simulink model "mpu6050 Simulink"  (R2025b)
settings: Solver=VariableStepAuto  StartTime=0.0  StopTime=10.0  RelTol=1e-3
PreLoadFcn:
  | Parameters_Flight_Firmware
undefined symbols (not defined in the file): Liftoff_threshold, threshold_sigma, Time
libraries: arduinolib x2, arduinosensorlib x1

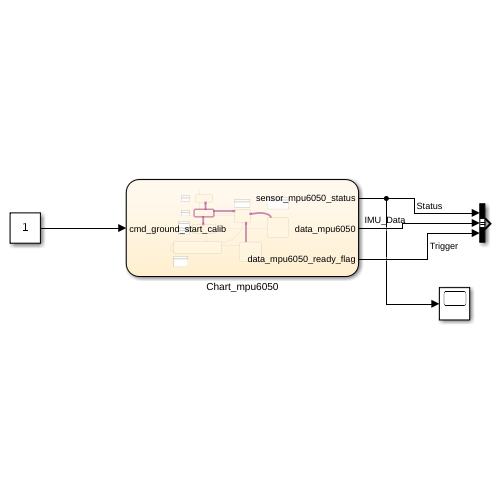
[thumbnail: Simulink's stored preview of the top-level diagram]
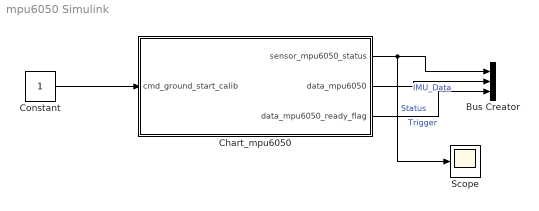
== system mpu6050 Simulink ==
  Bus Creator : BusCreator  Inputs=3
  Chart_mpu6050 : Stateflow chart  TreatAsAtomicUnit=on
  Constant : Constant
  Scope : Scope
  wires:
  Constant/1 -> Chart_mpu6050/1(cmd_ground_start_calib)
  Chart_mpu6050/1(sensor_mpu6050_status) -> Scope/1, Bus Creator/1  "Status"
  Chart_mpu6050/2(data_mpu6050) -> Bus Creator/2  "IMU_Data"
  Chart_mpu6050/3(data_mpu6050_ready_flag) -> Bus Creator/3  "Trigger"

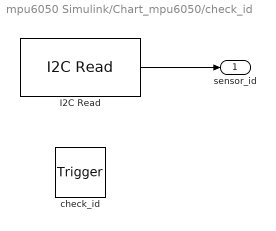
== system mpu6050 Simulink/Chart_mpu6050/check_id ==
  check_id : TriggerPort  TriggerType=function-call  VariantControl=(inherit)
      settings: CopyFcn=Stateflow.SLINSF.SimulinkMan.removeBlockPreDeleteFcn  PreDeleteFcn=Stateflow.SLINSF.SimulinkMan.unsafePredeleteFcn
  I2C Read : arduinolib/I2C Read  I2CModule=0  Mode=Master  SlaveAddress=0X68  SlaveByteOrder=BigEndian  Direction=Receiver  RegisterAddressMode=on  RegisterAddress=0X75  SlaveDataType=uint8  DataLength=1  NoAck=off  RepeatedStart=off  OutputStatus=off  blockPlatform=ARDUINO  SampleTime=-1
  sensor_id : Outport
  wires:
  I2C Read/1 -> sensor_id/1

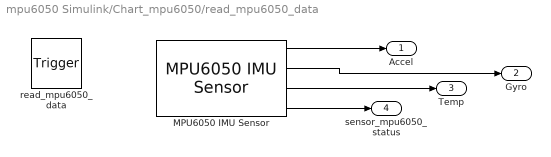
== system mpu6050 Simulink/Chart_mpu6050/read_mpu6050_data ==
  read_mpu6050_data : TriggerPort  TriggerType=function-call  VariantControl=(inherit)
      settings: CopyFcn=Stateflow.SLINSF.SimulinkMan.removeBlockPreDeleteFcn  PreDeleteFcn=Stateflow.SLINSF.SimulinkMan.unsafePredeleteFcn
  MPU6050 IMU Sensor : arduinosensorlib/MPU6050 IMU Sensor  I2CModule=0  SlaveAddress=0x68  Accel=on  AngularRate=on  Temperature=on  Status=on  Timestamp=off  EulerAngles=off  Quat=off  AccelRange=16G  GyroRange=2000 dps  DmpOdr=200 Hz  Dlpf=Accelerometer: 44Hz, Gyroscope: 42Hz  spf=1  SampleTime=-1  QueueSizeFactor=1
  Accel : Outport  OutDataTypeStr=double  PortDimensions=3
  Gyro : Outport  Port=2  OutDataTypeStr=double  PortDimensions=3
  Temp : Outport  Port=3  OutDataTypeStr=double  PortDimensions=1
  sensor_mpu6050_status : Outport  Port=4  OutDataTypeStr=uint8  PortDimensions=1
  wires:
  MPU6050 IMU Sensor/1 -> Accel/1
  MPU6050 IMU Sensor/2 -> Gyro/1
  MPU6050 IMU Sensor/3 -> Temp/1
  MPU6050 IMU Sensor/4 -> sensor_mpu6050_status/1

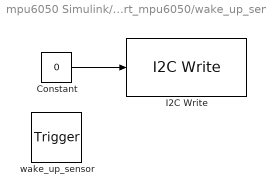
== system mpu6050 Simulink/Chart_mpu6050/wake_up_sensor ==
  wake_up_sensor : TriggerPort  TriggerType=function-call  VariantControl=(inherit)
      settings: CopyFcn=Stateflow.SLINSF.SimulinkMan.removeBlockPreDeleteFcn  PreDeleteFcn=Stateflow.SLINSF.SimulinkMan.unsafePredeleteFcn
  Constant : Constant  Value=0
  I2C Write : arduinolib/I2C Write  I2CModule=0  Mode=Master  SlaveAddress=0x68  SlaveByteOrder=BigEndian  Direction=Transmitter  RegisterAddressMode=on  RegisterAddress=0x6B  SlaveDataType=uint8  DataLength=1  NoAck=off  RepeatedStart=off  OutputStatus=off  blockPlatform=ARDUINO
  wires:
  Constant/1 -> I2C Write/1

== stateflow chart mpu6050 Simulink/Chart_mpu6050 ==
  state Power_on
    // Inizializza porte I2C
    entry: wake_up_sensor();
    delay_counter = 0;
    calib_done = false;
    during: delay_counter++;
  state wake_up_sensor [function]
  state [Accel, Gyro, Temp, sensor_mpu6050_status] = read_mpu6050_data [function]
  state Fault
    system_ready = false;
    entry: sensor_mpu6050_status = -1; // fault identity check - calibrazione fallita - Errore/Recupero
    during:
    data_mpu6050[0] = -999;
    data_mpu6050[1] = -999;
    data_mpu6050[2] = -999;
    data_mpu6050[3] = -999;
    data_mpu6050[4] = -999;
    data_mpu6050[5] = -999;
  state Sanity_Check
    entry: id_val = check_id();
    sensor_mpu6050_status = 0; // Verifica identità sensore
  state sensor_id = check_id [function]
  state Data_mpu6050_Acquisition_Raw
    entry: sensor_mpu6050_status = 3; // Sensore non calibrato - dati raw(dati grezzi)
    during: [Accel, Gyro, Temp, sensor_mpu6050_status] = read_mpu6050_data(); // Chiamata alla funzione che aggiorna le variabili locali-output per leggere i dati Raw
    // Assegnazione ai 7 slot del vettore data_mpu6050
    // Accelerazione Raw
    data_mpu6050[0] = Accel[0];
    data_mpu6050[1] = Accel[1];
    data_mpu6050[2] = Accel[2];
    // Giroscopio Raw
    data_mpu6050[3] = Gyro[0];
    data_mpu6050[4] = Gyro[1];
    data_mpu6050[5] = Gyro[2];
    // Stato Sensore mpu6050
    data_mpu6050[6] = sensor_mpu6050_status;
    data_mpu6050_ready_flag = true; // Alza il flag per il logger - via libera per la registrazione dei dati su SD
    exit: data_mpu6050_ready_flag = false; // Abbassa il flag quando esci da Data_mpu6050_Acquisition
  state Standby
    entry: system_ready = true; //Stato di attesa
    during: [Accel, Gyro, Temp, sensor_mpu6050_status] = read_mpu6050_data(); // Funzione che legge i dati grezzi dal sensore
    vibration = calc_vibration(Accel); // Calcolo la vibrazione dovuta all'accelerazione
    Az = accel_z(Accel); // Estraggo componente Z di Accel
  state Calibrating
    entry: sensor_mpu6050_status = 1; // Calibrazione del Sensore in Corso
    Reset = 1; // Al primo ingresso resettiamo la funzione Reset
    during: [Accel, Gyro, Temp, sensor_mpu6050_status] = read_mpu6050_data(); // Funzione che legge i dati grezzi dal sensore
    [mean_val, sigma, calib_done, under_threshold] = calib(Accel, Gyro, Reset, threshold_sigma)
    Reset = 0; // Dopo il primo ciclo mettiamo a 0 per continuare l'accumulo
    // Alla fine variabile calibration_done = true e mean_val == bias_val
  state Data_mpu6050_Acquisition
    entry: sensor_mpu6050_status = 2; // Stato Operativo - dati calibrati pronti per logging
    during: [Accel, Gyro, Temp, sensor_mpu6050_status] = read_mpu6050_data(); // Chiamata alla funzione che aggiorna le variabili locali-output per leggere i dati Raw
    // Assegnazione ai 7 slot del vettore data_mpu6050 sottraendo lo Zero-Bias
    // Accelerazione corretta
    data_mpu6050[0] = Accel[0] - bias_val[0];
    data_mpu6050[1] = Accel[1] - bias_val[1];
    data_mpu6050[2] = Accel[2] - bias_val[2];
    // Giroscopio corretta
    data_mpu6050[3] = Gyro[0] - bias_val[3];
    data_mpu6050[4] = Gyro[1] - bias_val[4];
    data_mpu6050[5] = Gyro[2] - bias_val[5];
    // Stato Sensore mpu6050
    data_mpu6050[6] = sensor_mpu6050_status;
    data_mpu6050_ready_flag = true; // Alza il flag per il logger - via libera per la registrazione dei dati su SD
    exit: data_mpu6050_ready_flag = false; // Abbassa il flag quando esci da Data_mpu6050_Acquisition
  (default) -> Power_on : {fail_count = 0;}
  Power_on -> Sanity_Check : [delay_counter >= 100]{fail_count = 0;}
  Sanity_Check -> Power_on [order 2] : [id_val != 104 && fail_count < 5] {fail_count = fail_count + 1;}
  Sanity_Check -> Fault [order 3] : [id_val != 104]
  Data_mpu6050_Acquisition -> Fault : [!recovery(id_val, sensor_mpu6050_status)]
  Fault -> Sanity_Check [order 1] : [fail_count < 100]{fail_count++;}
  Data_mpu6050_Acquisition_Raw -> Fault : [!recovery(id_val, sensor_mpu6050_status)]
  Fault -> Sanity_Check [order 2] : [fail_count >= 100]{fail_count = 0;}
  Sanity_Check -> Standby [order 1] : [id_val == 104]{fail_count = 0;}
  Calibrating -> Fault [order 2] : [check_id() != 104]
  Standby -> Data_mpu6050_Acquisition_Raw [order 2] : [duration(Az > Liftoff_threshold) > Time]
  Standby -> Calibrating [order 1] : [cmd_ground_start_calib == 1 && duration(vibration < Liftoff_threshold) > Time]
  Calibrating -> Calibrating [order 3] : [calib_done && !under_threshold]{Reset = 1;}
  Calibrating -> Data_mpu6050_Acquisition [order 1] : [calib_done && under_threshold]{bias_val = mean_val;}
  data: value_id function_input double; status function_input double; sanity_check function_output boolean; Accel function_output double size=3; Gyro function_output double size=3; Temp function_output double size=1; sensor_mpu6050_status function_output uint8 size=1; sensor_id function_output; oscillation function_output double; acc function_input double size=3; Acc function_input double size=3; az function_output double size=1; Acceleration function_input double size=3; Gyroscope function_input double size=3; reset function_input double; mean_value function_output double size=6; Sigma function_output double size=6; calibration_done function_output boolean; threshold_Sigma function_input double; Under_threshold function_output boolean; fail_count local uint8 size=1 =0; id_val local uint8 size=1; delay_counter local uint16; cmd_ground_start_calib input double; current_val local double size=6; sum_x local double size=6; sum_x2 local double size=6; variance local double size=6; sigma local double size=6; mean_val local double size=6; threshold_sigma parameter; Time parameter; Liftoff_threshold parameter; sensor_mpu6050_status output boolean size=1; data_mpu6050 output double size=7; data_mpu6050_ready_flag output boolean size=1; system_ready local boolean; Gyro local double size=3; Temp local int16 size=1; vibration local double =0; Accel local double size=3; Az local double size=1 =0; Reset local double; bias_val local double size=6; calib_done local double; under_threshold local boolean
  function sanity_check = recovery(value_id, status):
    | function sanity_check = recovery(value_id, status)
    | % value_id = check_id() - valore letto dal registro WHO_AM_I
    | % sensor_mpu6050_status - stato in cui mi trovo nella chart
    | 
    |  sanity_check = true; % Stato di Default sempre vero
    | 
    |  switch status
    |      case 0 % Verifica identità sensore
    |      case 1 % Calibrazione del sensore in corso
    |          if value_id ~= 104
    |              sanity_check = false;
    |          end
    |      case 2 % Stato Operativo - dati calibrati pronti per il logging
    |          if value_id ~= 104
    |              sanity_check = false;
    |          end
    |      case 3 % Sensore non calibrato - dati raw(grezzi)
    |          if value_id ~= 104
    |              sanity_check = false;
    |          end
    |      case 4 % fault identity check oppure calibrazione fallita- Errore/Recupero
    |          if value_id ~= 104
    |              sanity_check = false;
    |          end
    |      otherwise
    |          sanity_check = false;
    |  end
    | end
  function oscillation = calc_vibration(acc):
    | function oscillation = calc_vibration(acc)
    | % Funzione che calcola l'intensità del vettore accelerazione [ax, ay, az]
    | % acc: variabile Locale della variabile Accel in uscita dal sensore
    | % oscillation: variabile Locale della variabile vibration
    |  
    |     Accel_m = norm(acc); % Calcolo la norma euclidea del vettore accelerazione
    |     
    |     gravity = 9.81; % accelerazione di gravità in m/s^2 altrimenti usare 1 se in unità g
    |     
    |     oscillation = abs(Accel_m - gravity); % Calcola il valore assoluto
    | end
  function az = accel_z(Acc):
    | function az = accel_z(Acc)
    | % Funzione che estrae l'accelerazione lungo l'asse Z
    | % az: variabile Locale della variabile Az - componente lungo Z
    | % Acc: variabile Locale della variabile Accel vettore [ax, ay, az]
    |     az = Acc(2); % Prendo la componente lungo l'asse Z
    | end
  function [mean_value, Sigma, calibration_done, Under_threshold] = calib(Acceleration, Gyroscope, reset, threshold_Sigma):
    | function [mean_value, Sigma, calibration_done, Under_threshold] = calib(Acceleration, Gyroscope, reset, threshold_Sigma)
    | % Funzione che opera una Calibrazione Statica su 500 campioni per il calcolo dello Zero-Bias
    | % mean_value: variabile Locale della variabile mean_val, indica la media sui 500 campioni
    | % Sigma: variabile Locale della variabile sigma, indica la deviazione standard
    | % Calibration_done: variabile Locale della variabile calib_done 
    | % Under_threshold: variabile Locale della variabile under_threshold - flag che indica se la calibrazione è affidabile
    | % Acceleration: variabile Locale della variabile Accel [ax,ay,az]
    | % Gyroscope: variabile Locale della variabile Gyro
    | % reset: variabile Locale della variabile Reset
    | %threhsold_Sigma: variabile Locale della variabile threhsold_sigma che indica la soglia di tolleranza  
    | 
    | 
    | % Dichiarazioni delle variabili che mantengono il valore in memoria (accumulatori)
    |    persistent sum_x sum_x2 calib_count;
    | 
    |    % Inizializzazione: azzera i Buffer al primo avvio
    |    if isempty(calib_count) || reset
    |        sum_x = zeros(6,1);
    |        sum_x2 = zeros(6,1);
    |        calib_count = 0;
    |    end
    | 
    |    % Pre-Inizializzazione Ouput
    |    calibration_done = false; 
    |    mean_value = zeros(6,1); 
    |    Sigma = zeros(6,1);
    | 
    |    if calib_count < 500
    |        current_val = [Acceleration; Gyroscope];
    |        sum_x = sum_x + current_val;
    |        sum_x2 = sum_x2 + (current_val.*current_val);
    |        calib_count = calib_count + 1;
    |    end
    | 
    |    Under_threshold = false; % Default
    |    % Quando arrivo a 500 campioni, calcola risultato finale
    |    if calib_count == 500
    |        mean_value = sum_x / 500; % Calcolo della Media Aritmetica
    |        variance = (sum_x2 / 500) - (mean_value.*mean_value); % Calcolo della Varianza
    |        Sigma = sqrt(max(variance,0)); % Calcolo della Deviazione Standard
    |        calibration_done = true;
    |        Under_threshold = all(Sigma < threshold_Sigma);
    |    end
    | end
